simulink model "DC_pos_22"  (R2024a)
settings: Solver=ode5  StartTime=0.0  StopTime=Tf  FixedStep=Ts  RelTol=1e-3
undefined symbols (not defined in the file): A, B, freq, Ki, Kp, Ref
libraries: fuzblock x1
settings Model: Creator=ashaw  LastModifiedBy=Claudia Yasar
settings DataIOCC: ReturnWorkspaceOutputs=off
settings DebuggingCC: AlgebraicLoopMsg=none  ArtificialAlgebraicLoopMsg=none  OperatingPointInterfaceChecksumMismatchMsg=none
settings RTWCC: GPUComputeCapability=3.5

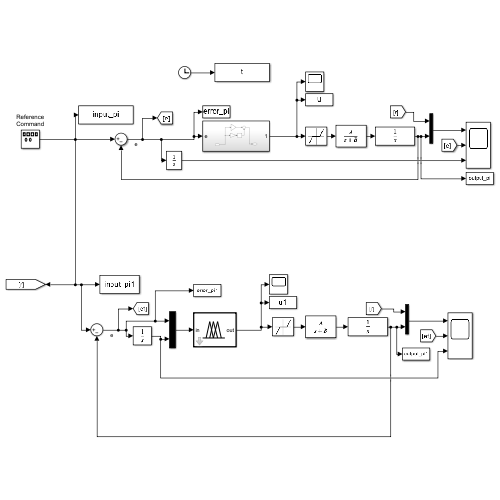
[thumbnail: Simulink's stored preview of the top-level diagram]
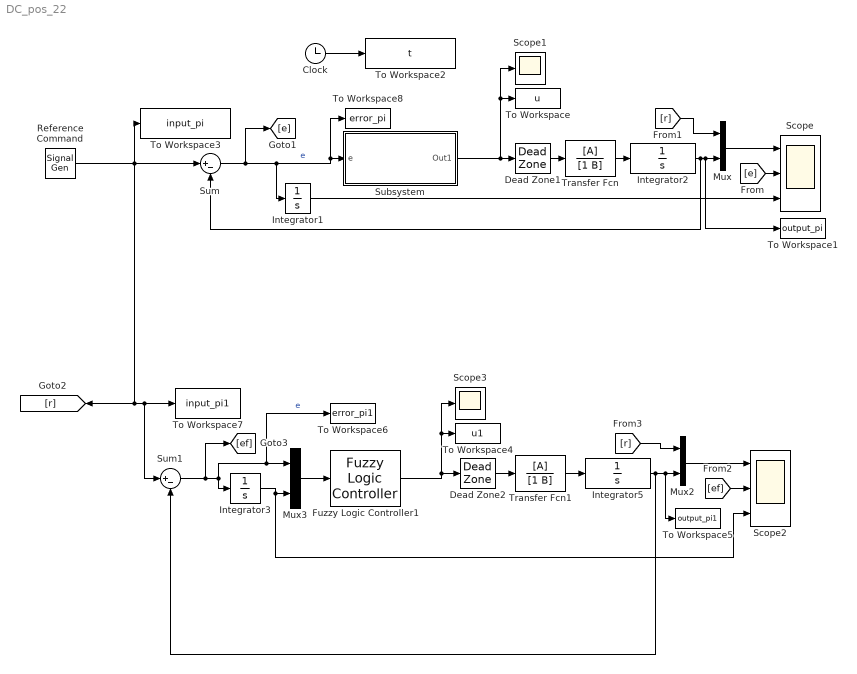
== system DC_pos_22 ==
  Clock : Clock
  Dead Zone1 : DeadZone  LowerValue=-0.05  UpperValue=0.05
  Dead Zone2 : DeadZone  LowerValue=-0.05  UpperValue=0.05
  Fuzzy Logic Controller1 : fuzblock/Fuzzy Logic  Controller  FIS=fis  OutputSampleNumber=101  DataType=double  FuzzifiedInputs=off  RuleFiringStrengths=off  RuleOutputs=off  AggregatedOutputs=off  SimulateUsing=Interpreted execution  OutOfRangeInputValueMessage=warning  NoRuleFiredMessage=warning  EmptyOutputFuzzySetMessage=warning
  Integrator{1..3,5} (4 alike) : Integrator
  Mux : Mux  Inputs=2
  Mux2 : Mux  Inputs=2
  Mux3 : Mux  Inputs=2
  Reference Command : SignalGenerator  WaveForm=square  Amplitude=Ref  Frequency=freq  Units=rad/sec
  Scope : Scope  NumInputPorts=3
  Scope1 : Scope
  Scope2 : Scope  NumInputPorts=3
  Scope3 : Scope
  Subsystem : Subsystem
  Sum : Sum  Inputs=|+-
  Sum1 : Sum  Inputs=|+-
  To Workspace : ToWorkspace  VariableName=u  SampleTime=-1
      settings: Save2DSignal=2-D array (concatenate along first dimension)
  To Workspace1 : ToWorkspace  VariableName=output_pi  SampleTime=-1
      settings: Save2DSignal=2-D array (concatenate along first dimension)
  To Workspace2 : ToWorkspace  VariableName=t  SampleTime=-1
  To Workspace3 : ToWorkspace  VariableName=input_pi  SampleTime=-1
  To Workspace4 : ToWorkspace  VariableName=u1  SampleTime=-1
      settings: Save2DSignal=2-D array (concatenate along first dimension)
  To Workspace5 : ToWorkspace  VariableName=output_pi1  SampleTime=-1
      settings: Save2DSignal=2-D array (concatenate along first dimension)
  To Workspace6 : ToWorkspace  VariableName=error_pi1  SampleTime=-1
      settings: Save2DSignal=2-D array (concatenate along first dimension)
  To Workspace7 : ToWorkspace  VariableName=input_pi1  SampleTime=-1
  To Workspace8 : ToWorkspace  VariableName=error_pi  SampleTime=-1
      settings: Save2DSignal=2-D array (concatenate along first dimension)
  Transfer Fcn : TransferFcn  Numerator=[A]  Denominator=[1 B]
  Transfer Fcn1 : TransferFcn  Numerator=[A]  Denominator=[1 B]
  wires:
  Sum/1 -> [e], To Workspace8/1, Subsystem/1(e), Integrator1/1  "e"
  Mux/1 -> Scope/1
  Integrator1/1 -> Scope/3
  [e] -> Scope/2
  [r] -> Mux/1
  Clock/1 -> To Workspace2/1
  Transfer Fcn/1 -> Integrator2/1
  Integrator2/1 -> Sum/2, To Workspace1/1, Mux/2
  Dead Zone1/1 -> Transfer Fcn/1
  Subsystem/1(Out1) -> Scope1/1, To Workspace/1, Dead Zone1/1
  Dead Zone2/1 -> Transfer Fcn1/1
  Fuzzy Logic Controller1/1 -> Scope3/1, To Workspace4/1, Dead Zone2/1
  Sum1/1 -> [ef], To Workspace6/1, Mux3/1, Integrator3/1  "e"
  Mux3/1 -> Fuzzy Logic Controller1/1
  Transfer Fcn1/1 -> Integrator5/1
  Mux2/1 -> Scope2/1
  [ef] -> Scope2/2
  [r] -> Mux2/1
  Integrator3/1 -> Mux3/2, Scope2/3
  Reference Command/1 -> To Workspace3/1, Sum1/1, To Workspace7/1, [r], Sum/1
  Integrator5/1 -> To Workspace5/1, Mux2/2, Sum1/2

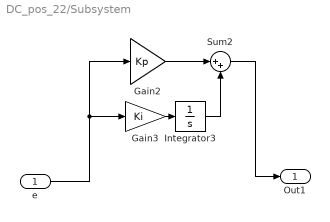
== system DC_pos_22/Subsystem ==
  e : Inport
  Gain2 : Gain  Gain=Kp
  Gain3 : Gain  Gain=Ki
  Integrator3 : Integrator
  Sum2 : Sum  Inputs=|++
  Out1 : Outport
  wires:
  e/1 -> Gain2/1, Gain3/1
  Gain3/1 -> Integrator3/1
  Integrator3/1 -> Sum2/2
  Gain2/1 -> Sum2/1
  Sum2/1 -> Out1/1
